simulink model "Predefined_time_v2"  (R2022a)
settings: Solver=ode8  StartTime=0  StopTime=1  FixedStep=1e-5  RelTol=1e-5
values from neighbouring files (symbols this model uses):
  order = 0.95    [predefined_time_M.m]
  phi_1 = (n*pi)/(4*Tc)    (= 47.1238898038)    [predefined_time_M.m]
  phi_2 = pi/(4*Tc)    (= 3.92699081699)    [predefined_time_M.m]
  phi_3 = (n*pi)/(4*Tc)    (= 47.1238898038)    [predefined_time_M.m]
  phi_4 = pi/(4*Tc)    (= 3.92699081699)    [predefined_time_M.m]
undefined symbols (not defined in the file or in its folder): phi_5, phi_6
libraries: cstblocks x32
(part 1 of 2)
settings Model: SimulationMode=accelerator  Creator=WIT531  LastModifiedBy=WIT531
settings SolverCC: ZeroCrossAlgorithm=Adaptive  EnableFixedStepZeroCrossing=on
settings DataIOCC: SaveFormat=Array  SaveOutput=off  SignalLogging=off  DSMLogging=off  SaveTime=off  ReturnWorkspaceOutputs=off  TimeSaveName=e2312tout  OutputSaveName=e2312
settings OptimizationCC: DefaultParameterBehavior=Inlined  EnhancedBackFolding=on  PassReuseOutputArgsAs=Individual arguments  ZeroExternalMemoryAtStartup=off  ZeroInternalMemoryAtStartup=off  InitFltsAndDblsToZero=on  OptimizeBlockOrder=speed  DifferentSizesBufferReuse=on  OptimizationCustomize=off  EfficientTunableParamExpr=on
settings DebuggingCC: ParameterTunabilityLossMsg=error
settings HardwareCC: ProdLongLongMode=on  TargetLongLongMode=on
settings SFSimCC: MATLABDynamicMemAlloc=off  SimTargetLang=C++
settings RTWCC: SystemTargetFile=ert.tlc  TemplateMakefile=ert_default_tmf  TargetLang=C++
settings CodeAppCC: ForceParamTrailComments=on  IgnoreCustomStorageClasses=off  OperatorAnnotations=on  SimulinkDataObjDesc=on  SFDataObjDesc=on  InsertBlockDesc=on
settings ERTTargetCC: TargetLangStandard=C++11 (ISO)  GenerateSampleERTMain=on  CodeInterfacePackaging=C++ class  InlinedParameterPlacement=NonHierarchical  RootIOFormat=Structure reference  ERTCustomFileTemplate=example_file_process.tlc

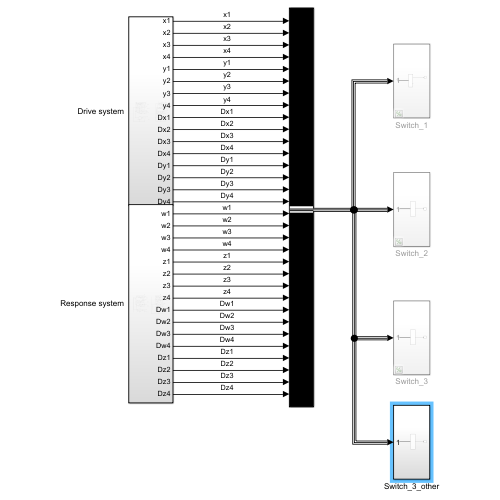
[thumbnail: Simulink's stored preview of the top-level diagram]
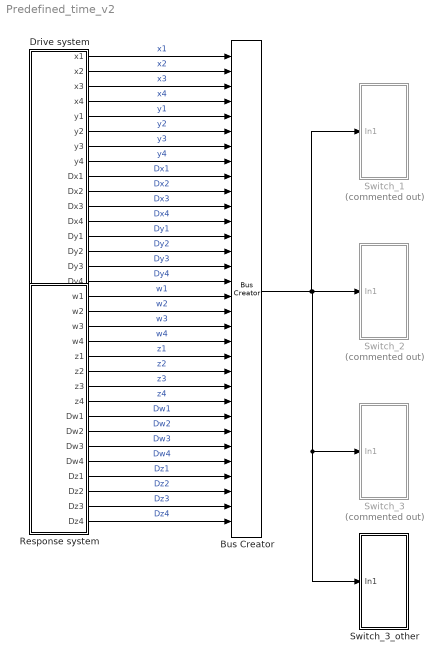
== system Predefined_time_v2 ==
  Bus Creator : BusCreator  Inputs=32
  Drive system : Subsystem
  Response system : Subsystem
  Switch_1 : Subsystem  Commented=on
  Switch_2 : Subsystem  Commented=on
  Switch_3 : Subsystem  Commented=on
  Switch_3_other : Subsystem
  wires:
  Bus Creator/1 -> Switch_3_other/1(In1), Switch_3/1(In1), Switch_2/1(In1), Switch_1/1(In1)
  Drive system/1(x1) -> Bus Creator/1  "x1"
  Drive system/2(x2) -> Bus Creator/2  "x2"
  Drive system/3(x3) -> Bus Creator/3  "x3"
  Drive system/4(x4) -> Bus Creator/4  "x4"
  Drive system/5(y1) -> Bus Creator/5  "y1"
  Drive system/6(y2) -> Bus Creator/6  "y2"
  Drive system/7(y3) -> Bus Creator/7  "y3"
  Drive system/8(y4) -> Bus Creator/8  "y4"
  Drive system/9(Dx1) -> Bus Creator/9  "Dx1"
  Drive system/10(Dx2) -> Bus Creator/10  "Dx2"
  Drive system/11(Dx3) -> Bus Creator/11  "Dx3"
  Drive system/12(Dx4) -> Bus Creator/12  "Dx4"
  Drive system/13(Dy1) -> Bus Creator/13  "Dy1"
  Drive system/14(Dy2) -> Bus Creator/14  "Dy2"
  Drive system/15(Dy3) -> Bus Creator/15  "Dy3"
  Drive system/16(Dy4) -> Bus Creator/16  "Dy4"
  Response system/9(Dw1) -> Bus Creator/25  "Dw1"
  Response system/10(Dw2) -> Bus Creator/26  "Dw2"
  Response system/11(Dw3) -> Bus Creator/27  "Dw3"
  Response system/12(Dw4) -> Bus Creator/28  "Dw4"
  Response system/13(Dz1) -> Bus Creator/29  "Dz1"
  Response system/14(Dz2) -> Bus Creator/30  "Dz2"
  Response system/15(Dz3) -> Bus Creator/31  "Dz3"
  Response system/16(Dz4) -> Bus Creator/32  "Dz4"
  Response system/1(w1) -> Bus Creator/17  "w1"
  Response system/2(w2) -> Bus Creator/18  "w2"
  Response system/3(w3) -> Bus Creator/19  "w3"
  Response system/4(w4) -> Bus Creator/20  "w4"
  Response system/5(z1) -> Bus Creator/21  "z1"
  Response system/6(z2) -> Bus Creator/22  "z2"
  Response system/7(z3) -> Bus Creator/23  "z3"
  Response system/8(z4) -> Bus Creator/24  "z4"

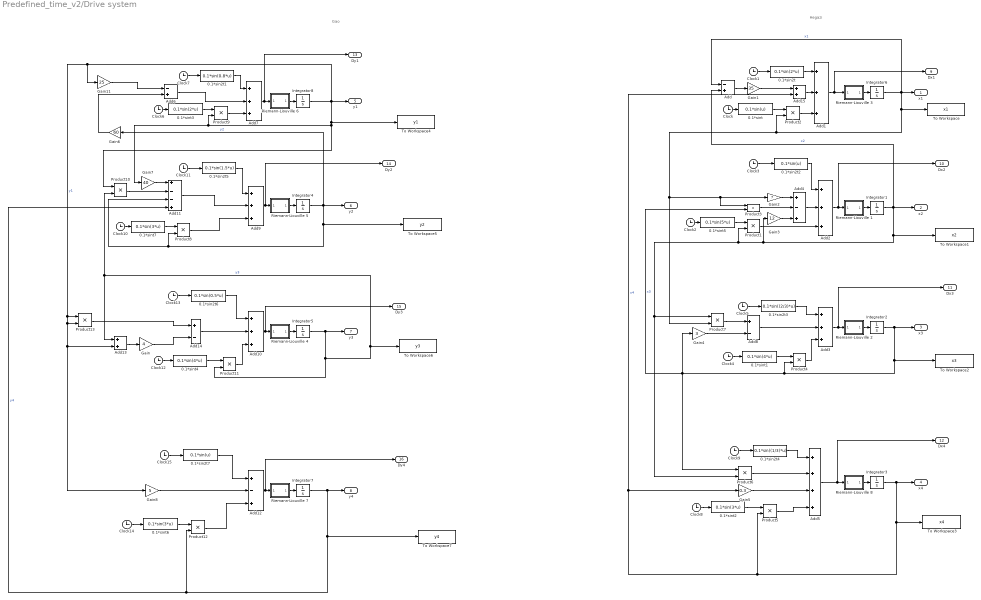
== system Predefined_time_v2/Drive system ==
  note: Gao
  note: Hegazi
  0.1*sin2t : MATLABFcn  MATLABFcn=0.1*sin(2*u)
  0.1*sin2t1 : MATLABFcn  MATLABFcn=0.1*sin(0.8*u)
  0.1*sin2t2 : MATLABFcn  MATLABFcn=0.1*sin(u)
  0.1*sin2t3 : MATLABFcn  MATLABFcn=0.1*sin((2/3)*u)
  0.1*sin2t4 : MATLABFcn  MATLABFcn=0.1*sin((1/3)*u)
  0.1*sin2t5 : MATLABFcn  MATLABFcn=0.1*sin(1.5*u)
  0.1*sin2t6 : MATLABFcn  MATLABFcn=0.1*sin(0.5*u)
  0.1*sin2t7 : MATLABFcn  MATLABFcn=0.1*sin(u)
  0.1*sint : MATLABFcn  MATLABFcn=0.1*sin(u)
  0.1*sint1 : MATLABFcn  MATLABFcn=0.1*sin(4*u)
  0.1*sint2 : MATLABFcn  MATLABFcn=0.1*sin(3*u)
  0.1*sint3 : MATLABFcn  MATLABFcn=0.1*sin(2*u)
  0.1*sint4 : MATLABFcn  MATLABFcn=0.1*sin(4*u)
  0.1*sint5 : MATLABFcn  MATLABFcn=0.1*sin(5*u)
  0.1*sint6 : MATLABFcn  MATLABFcn=0.1*sin(3*u)
  0.1*sint7 : MATLABFcn  MATLABFcn=0.1*sin(3*u)
  Add : Sum  Inputs=-+
  Add{1..3,7,9..10} (6 alike) : Sum  Inputs=+++
  Add11 : Sum  Inputs=+--+
  Add12 : Sum  Inputs=+-+
  Add13 : Sum
  Add14 : Sum  Inputs=+-
  Add15 : Sum
  Add4 : Sum  Inputs=+-+
  Add5 : Sum  Inputs=++++
  Add6 : Sum  Inputs=-+
  Add8 : Sum  Inputs=+-
  Clock{,1..15} (16 alike) : Clock
  Gain : Gain  Gain=4
  Gain1 : Gain  Gain=35
  Gain11 : Gain  Gain=25
  Gain2 : Gain  Gain=7
  Gain3 : Gain  Gain=12
  Gain4 : Gain  Gain=3
  Gain5 : Gain  Gain=0.3
  Gain6 : Gain  Gain=60
  Gain7 : Gain  Gain=40
  Gain8 : Gain  Gain=5
  Integrator{1..3,6,8} (5 alike) : Integrator  InitialCondition=10
  Integrator4 : Integrator  InitialCondition=12
  Integrator5 : Integrator  InitialCondition=15
  Integrator7 : Integrator  InitialCondition=12
  Product{1..13} (13 alike) : Product
  Riemann-Liouville 1 : Subsystem  mask{gam=1-order, ww=[1e-3, 1e3], n=5, kF1=off, kF=Oustaloup filter}
      mask prompts: gam "Derivative order gamma"; ww "Frequency range [wb,wh]"; n "Apprixmation order"; kF1 "Is a low-pass filter required?"; kF "Filter type"
      mask init:
      | wb=ww(1); wh=ww(2); 
      | if isnumeric(gam), str=['{\its}^{' num2str(gam) '}']; 
      | else, str='{\its}^{\gamma}'; end
      | if kF==1, G=ousta_fod(gam,n,wb,wh);
      | elseif kF==2, G=new_fod(gam,n,wb,wh); 
      | else, G=matsuda_fod(gam,n,wb,wh); end
      | T=1/wh; if kF1==1, G=G*tf(1,[T 1]); end
      mask TypeOptions kF: Oustaloup filter | Modified Oustaloup filter | Matsuda-Fujii filter
      mask Display: disp(str,'texmode','on')
  Riemann-Liouville 2 : Subsystem  mask{gam=1-order, ww=[1e-3, 1e3], n=5, kF1=off, kF=Oustaloup filter}
      mask prompts: gam "Derivative order gamma"; ww "Frequency range [wb,wh]"; n "Apprixmation order"; kF1 "Is a low-pass filter required?"; kF "Filter type"
      mask init: same as Predefined_time_v2/Drive system/Riemann-Liouville 1
      mask TypeOptions kF: Oustaloup filter | Modified Oustaloup filter | Matsuda-Fujii filter
      mask Display: disp(str,'texmode','on')
  Riemann-Liouville 3 : Subsystem  mask{gam=1-order, ww=[1e-3, 1e3], n=5, kF1=off, kF=Oustaloup filter}
      mask prompts: gam "Derivative order gamma"; ww "Frequency range [wb,wh]"; n "Apprixmation order"; kF1 "Is a low-pass filter required?"; kF "Filter type"
      mask init: same as Predefined_time_v2/Drive system/Riemann-Liouville 1
      mask TypeOptions kF: Oustaloup filter | Modified Oustaloup filter | Matsuda-Fujii filter
      mask Display: disp(str,'texmode','on')
  Riemann-Liouville 4 : Subsystem  mask{gam=1-order, ww=[1e-3, 1e3], n=5, kF1=off, kF=Oustaloup filter}
      mask prompts: gam "Derivative order gamma"; ww "Frequency range [wb,wh]"; n "Apprixmation order"; kF1 "Is a low-pass filter required?"; kF "Filter type"
      mask init: same as Predefined_time_v2/Drive system/Riemann-Liouville 1
      mask TypeOptions kF: Oustaloup filter | Modified Oustaloup filter | Matsuda-Fujii filter
      mask Display: disp(str,'texmode','on')
  Riemann-Liouville 5 : Subsystem  mask{gam=1-order, ww=[1e-3, 1e3], n=5, kF1=off, kF=Oustaloup filter}
      mask prompts: gam "Derivative order gamma"; ww "Frequency range [wb,wh]"; n "Apprixmation order"; kF1 "Is a low-pass filter required?"; kF "Filter type"
      mask init: same as Predefined_time_v2/Drive system/Riemann-Liouville 1
      mask TypeOptions kF: Oustaloup filter | Modified Oustaloup filter | Matsuda-Fujii filter
      mask Display: disp(str,'texmode','on')
  Riemann-Liouville 6 : Subsystem  mask{gam=1-order, ww=[1e-3, 1e3], n=5, kF1=off, kF=Oustaloup filter}
      mask prompts: gam "Derivative order gamma"; ww "Frequency range [wb,wh]"; n "Apprixmation order"; kF1 "Is a low-pass filter required?"; kF "Filter type"
      mask init: same as Predefined_time_v2/Drive system/Riemann-Liouville 1
      mask TypeOptions kF: Oustaloup filter | Modified Oustaloup filter | Matsuda-Fujii filter
      mask Display: disp(str,'texmode','on')
  Riemann-Liouville 7 : Subsystem  mask{gam=1-order, ww=[1e-3, 1e3], n=5, kF1=off, kF=Oustaloup filter}
      mask prompts: gam "Derivative order gamma"; ww "Frequency range [wb,wh]"; n "Apprixmation order"; kF1 "Is a low-pass filter required?"; kF "Filter type"
      mask init: same as Predefined_time_v2/Drive system/Riemann-Liouville 1
      mask TypeOptions kF: Oustaloup filter | Modified Oustaloup filter | Matsuda-Fujii filter
      mask Display: disp(str,'texmode','on')
  Riemann-Liouville 8 : Subsystem  mask{gam=1-order, ww=[1e-3, 1e3], n=5, kF1=off, kF=Oustaloup filter}
      mask prompts: gam "Derivative order gamma"; ww "Frequency range [wb,wh]"; n "Apprixmation order"; kF1 "Is a low-pass filter required?"; kF "Filter type"
      mask init: same as Predefined_time_v2/Drive system/Riemann-Liouville 1
      mask TypeOptions kF: Oustaloup filter | Modified Oustaloup filter | Matsuda-Fujii filter
      mask Display: disp(str,'texmode','on')
  To Workspace : ToWorkspace  VariableName=x1  SaveFormat=Timeseries  SampleTime=-1
  To Workspace1 : ToWorkspace  VariableName=x2  SaveFormat=Timeseries  SampleTime=-1
  To Workspace2 : ToWorkspace  VariableName=x3  SaveFormat=Timeseries  SampleTime=-1
  To Workspace3 : ToWorkspace  VariableName=x4  SaveFormat=Timeseries  SampleTime=-1
  To Workspace4 : ToWorkspace  VariableName=y1  SaveFormat=Timeseries  SampleTime=-1
  To Workspace5 : ToWorkspace  VariableName=y2  SaveFormat=Timeseries  SampleTime=-1
  To Workspace6 : ToWorkspace  VariableName=y3  SaveFormat=Timeseries  SampleTime=-1
  To Workspace7 : ToWorkspace  VariableName=y4  SaveFormat=Timeseries  SampleTime=-1
  x1 : Outport
  x2 : Outport  Port=2
  x3 : Outport  Port=3
  x4 : Outport  Port=4
  y1 : Outport  Port=5
  y2 : Outport  Port=6
  y3 : Outport  Port=7
  y4 : Outport  Port=8
  Dx1 : Outport  Port=9
  Dx2 : Outport  Port=10
  Dx3 : Outport  Port=11
  Dx4 : Outport  Port=12
  Dy1 : Outport  Port=13
  Dy2 : Outport  Port=14
  Dy3 : Outport  Port=15
  Dy4 : Outport  Port=16
  wires:
  Integrator6/1 -> Add/1, x1/1, To Workspace/1, Product2/2, Product7/2, Product3/1, Gain2/1  "x1"
  Add1/1 -> Riemann-Liouville 3/1(In1), Dx1/1
  0.1*sint/1 -> Product2/1
  Clock/1 -> 0.1*sint/1
  Clock1/1 -> 0.1*sin2t/1
  Add2/1 -> Riemann-Liouville 1/1(In1), Dx2/1
  Add/1 -> Gain1/1
  Gain1/1 -> Add15/1
  0.1*sint5/1 -> Product1/1
  Integrator1/1 -> Add/2, x2/1, To Workspace1/1, Product7/1, Product6/2, Product1/2, Gain3/1  "x2"
  Clock2/1 -> 0.1*sint5/1
  Clock3/1 -> 0.1*sin2t2/1
  Gain2/1 -> Add4/1
  Integrator2/1 -> To Workspace2/1, Product6/1, Gain4/1, Product3/2, Product4/2, x3/1  "x3"
  Add3/1 -> Riemann-Liouville 2/1(In1), Dx3/1
  Add4/1 -> Add2/2
  Add5/1 -> Riemann-Liouville 8/1(In1), Dx4/1
  Integrator3/1 -> To Workspace3/1, Gain5/1, Add15/2, Product5/2, x4/1  "x4"
  Clock4/1 -> 0.1*sint1/1
  0.1*sint1/1 -> Product4/1
  Add8/1 -> Add3/2
  Clock5/1 -> 0.1*sin2t3/1
  Product6/1 -> Add5/2
  Gain5/1 -> Add5/3
  Clock8/1 -> 0.1*sint2/1
  0.1*sint2/1 -> Product5/1
  Clock9/1 -> 0.1*sin2t4/1
  Product7/1 -> Add8/1
  Clock13/1 -> 0.1*sin2t6/1
  Clock12/1 -> 0.1*sint4/1
  Integrator7/1 -> To Workspace7/1, Add11/4, Product12/2, y4/1  "y4"
  Add12/1 -> Riemann-Liouville 7/1(In1), Dy4/1
  Add10/1 -> Riemann-Liouville 4/1(In1), Dy3/1
  Clock14/1 -> 0.1*sint6/1
  0.1*sint7/1 -> Product8/1
  Clock10/1 -> 0.1*sint7/1
  Clock7/1 -> 0.1*sin2t1/1
  0.1*sint3/1 -> Product9/1
  Clock11/1 -> 0.1*sin2t5/1
  Clock6/1 -> 0.1*sint3/1
  Integrator8/1 -> Gain11/1, Add13/2, Gain8/1, Product13/2, Product13/1, y1/1, To Workspace4/1, Product10/1, Gain7/1, Product9/2  "y1"
  Add6/1 -> Add7/2
  Integrator5/1 -> To Workspace6/1, Add13/1, Product10/2, Product11/2, y3/1  "y3"
  Add7/1 -> Riemann-Liouville 6/1(In1), Dy1/1
  0.1*sint4/1 -> Product11/1
  Clock15/1 -> 0.1*sin2t7/1
  0.1*sint6/1 -> Product12/1
  Add9/1 -> Riemann-Liouville 5/1(In1), Dy2/1
  Riemann-Liouville 7/1(Out1) -> Integrator7/1
  Add11/1 -> Add9/2
  Add13/1 -> Gain/1
  Product13/1 -> Add14/1
  Gain/1 -> Add14/2
  Add14/1 -> Add10/2
  Gain8/1 -> Add12/2
  Add15/1 -> Add1/2
  Product3/1 -> Add4/2
  Gain3/1 -> Add4/3
  Gain7/1 -> Add11/1
  Product10/1 -> Add11/2
  Integrator4/1 -> Gain6/1, To Workspace5/1, Add11/3, Product8/2, y2/1  "y2"
  Riemann-Liouville 6/1(Out1) -> Integrator8/1
  Riemann-Liouville 5/1(Out1) -> Integrator4/1
  Riemann-Liouville 4/1(Out1) -> Integrator5/1
  Riemann-Liouville 3/1(Out1) -> Integrator6/1
  Riemann-Liouville 1/1(Out1) -> Integrator1/1
  Riemann-Liouville 2/1(Out1) -> Integrator2/1
  Riemann-Liouville 8/1(Out1) -> Integrator3/1
  0.1*sin2t1/1 -> Add7/1
  Product9/1 -> Add7/3
  0.1*sin2t5/1 -> Add9/1
  Product8/1 -> Add9/3
  0.1*sin2t6/1 -> Add10/1
  Product11/1 -> Add10/3
  0.1*sin2t7/1 -> Add12/1
  Product12/1 -> Add12/3
  Product5/1 -> Add5/4
  0.1*sin2t4/1 -> Add5/1
  Product4/1 -> Add3/3
  0.1*sin2t3/1 -> Add3/1
  0.1*sin2t2/1 -> Add2/1
  Product1/1 -> Add2/3
  Product2/1 -> Add1/3
  0.1*sin2t/1 -> Add1/1
  Gain4/1 -> Add8/2
  Gain11/1 -> Add6/1
  Gain6/1 -> Add6/2

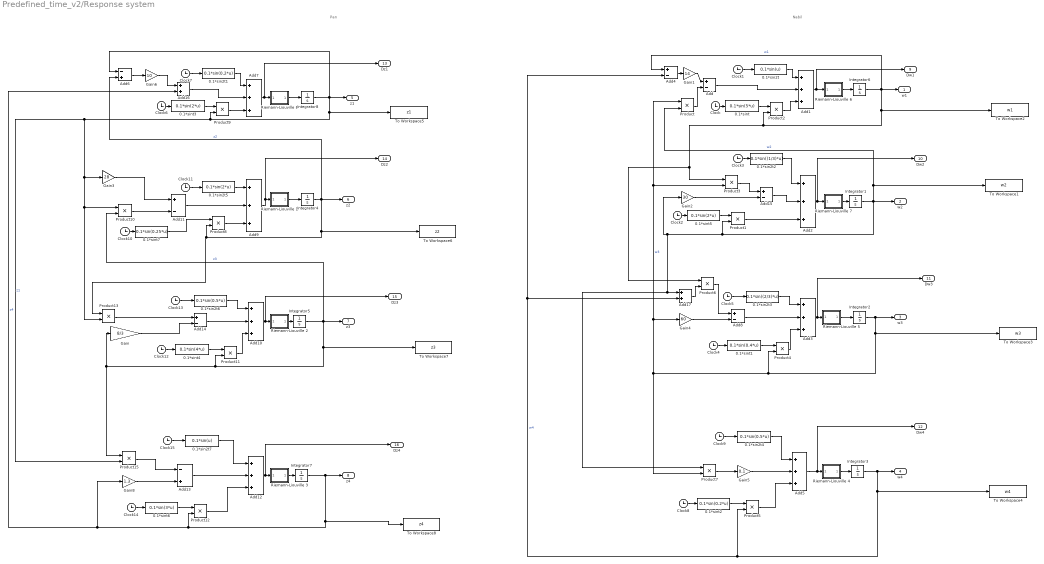
== system Predefined_time_v2/Response system ==
  note: Pan
  note: Nabil
  0.1*sin2t : MATLABFcn  MATLABFcn=0.1*sin(u)
  0.1*sin2t1 : MATLABFcn  MATLABFcn=0.1*sin(0.2*u)
  0.1*sin2t2 : MATLABFcn  MATLABFcn=0.1*sin((1/3)*u)
  0.1*sin2t3 : MATLABFcn  MATLABFcn=0.1*sin((2/3)*u)
  0.1*sin2t4 : MATLABFcn  MATLABFcn=0.1*sin(0.5*u)
  0.1*sin2t5 : MATLABFcn  MATLABFcn=0.1*sin(2*u)
  0.1*sin2t6 : MATLABFcn  MATLABFcn=0.1*sin(0.5*u)
  0.1*sin2t7 : MATLABFcn  MATLABFcn=0.1*sin(u)
  0.1*sint : MATLABFcn  MATLABFcn=0.1*sin(5*u)
  0.1*sint1 : MATLABFcn  MATLABFcn=0.1*sin(0.4*u)
  0.1*sint2 : MATLABFcn  MATLABFcn=0.1*sin(0.2*u)
  0.1*sint3 : MATLABFcn  MATLABFcn=0.1*sin(2*u)
  0.1*sint4 : MATLABFcn  MATLABFcn=0.1*sin(4*u)
  0.1*sint5 : MATLABFcn  MATLABFcn=0.1*sin(2*u)
  0.1*sint6 : MATLABFcn  MATLABFcn=0.1*sin(3*u)
  0.1*sint7 : MATLABFcn  MATLABFcn=0.1*sin(0.25*u)
  Add{,4,8,11,14..15} (6 alike) : Sum  Inputs=+-
  Add{1..3,5,7,9..10,12} (8 alike) : Sum  Inputs=+++
  Add13 : Sum  Inputs=-+
  Add16 : Sum
  Add17 : Sum
  Add6 : Sum  Inputs=-+
  Clock{,1..15} (16 alike) : Clock
  Gain : Gain  Gain=8/3
  Gain1 : Gain  Gain=14
  Gain2 : Gain  Gain=30
  Gain3 : Gain  Gain=28
  Gain4 : Gain  Gain=60
  Gain5 : Gain  Gain=0.1
  Gain6 : Gain  Gain=10
  Gain8 : Gain  Gain=1.3
  Integrator1 : Integrator  InitialCondition=14
  Integrator2 : Integrator  InitialCondition=12
  Integrator3 : Integrator  InitialCondition=13
  Integrator4 : Integrator  InitialCondition=3
  Integrator5 : Integrator  InitialCondition=16
  Integrator6 : Integrator  InitialCondition=21
  Integrator7 : Integrator  InitialCondition=17
  Integrator8 : Integrator  InitialCondition=15
  Product{,1..13,15} (15 alike) : Product
  Riemann-Liouville 1 : Subsystem  mask{gam=1-order, ww=[1e-3, 1e3], n=5, kF1=off, kF=Oustaloup filter}
      mask prompts: gam "Derivative order gamma"; ww "Frequency range [wb,wh]"; n "Apprixmation order"; kF1 "Is a low-pass filter required?"; kF "Filter type"
      mask init: same as Predefined_time_v2/Drive system/Riemann-Liouville 1
      mask TypeOptions kF: Oustaloup filter | Modified Oustaloup filter | Matsuda-Fujii filter
      mask Display: disp(str,'texmode','on')
  Riemann-Liouville 2 : Subsystem  mask{gam=1-order, ww=[1e-3, 1e3], n=5, kF1=off, kF=Oustaloup filter}
      mask prompts: gam "Derivative order gamma"; ww "Frequency range [wb,wh]"; n "Apprixmation order"; kF1 "Is a low-pass filter required?"; kF "Filter type"
      mask init: same as Predefined_time_v2/Drive system/Riemann-Liouville 1
      mask TypeOptions kF: Oustaloup filter | Modified Oustaloup filter | Matsuda-Fujii filter
      mask Display: disp(str,'texmode','on')
  Riemann-Liouville 3 : Subsystem  mask{gam=1-order, ww=[1e-3, 1e3], n=5, kF1=off, kF=Oustaloup filter}
      mask prompts: gam "Derivative order gamma"; ww "Frequency range [wb,wh]"; n "Apprixmation order"; kF1 "Is a low-pass filter required?"; kF "Filter type"
      mask init: same as Predefined_time_v2/Drive system/Riemann-Liouville 1
      mask TypeOptions kF: Oustaloup filter | Modified Oustaloup filter | Matsuda-Fujii filter
      mask Display: disp(str,'texmode','on')
  Riemann-Liouville 4 : Subsystem  mask{gam=1-order, ww=[1e-3, 1e3], n=5, kF1=off, kF=Oustaloup filter}
      mask prompts: gam "Derivative order gamma"; ww "Frequency range [wb,wh]"; n "Apprixmation order"; kF1 "Is a low-pass filter required?"; kF "Filter type"
      mask init: same as Predefined_time_v2/Drive system/Riemann-Liouville 1
      mask TypeOptions kF: Oustaloup filter | Modified Oustaloup filter | Matsuda-Fujii filter
      mask Display: disp(str,'texmode','on')
  Riemann-Liouville 5 : Subsystem  mask{gam=1-order, ww=[1e-3, 1e3], n=5, kF1=off, kF=Oustaloup filter}
      mask prompts: gam "Derivative order gamma"; ww "Frequency range [wb,wh]"; n "Apprixmation order"; kF1 "Is a low-pass filter required?"; kF "Filter type"
      mask init: same as Predefined_time_v2/Drive system/Riemann-Liouville 1
      mask TypeOptions kF: Oustaloup filter | Modified Oustaloup filter | Matsuda-Fujii filter
      mask Display: disp(str,'texmode','on')
  Riemann-Liouville 6 : Subsystem  mask{gam=1-order, ww=[1e-3, 1e3], n=5, kF1=off, kF=Oustaloup filter}
      mask prompts: gam "Derivative order gamma"; ww "Frequency range [wb,wh]"; n "Apprixmation order"; kF1 "Is a low-pass filter required?"; kF "Filter type"
      mask init: same as Predefined_time_v2/Drive system/Riemann-Liouville 1
      mask TypeOptions kF: Oustaloup filter | Modified Oustaloup filter | Matsuda-Fujii filter
      mask Display: disp(str,'texmode','on')
  Riemann-Liouville 7 : Subsystem  mask{gam=1-order, ww=[1e-3, 1e3], n=5, kF1=off, kF=Oustaloup filter}
      mask prompts: gam "Derivative order gamma"; ww "Frequency range [wb,wh]"; n "Apprixmation order"; kF1 "Is a low-pass filter required?"; kF "Filter type"
      mask init: same as Predefined_time_v2/Drive system/Riemann-Liouville 1
      mask TypeOptions kF: Oustaloup filter | Modified Oustaloup filter | Matsuda-Fujii filter
      mask Display: disp(str,'texmode','on')
  Riemann-Liouville 8 : Subsystem  mask{gam=1-order, ww=[1e-3, 1e3], n=5, kF1=off, kF=Oustaloup filter}
      mask prompts: gam "Derivative order gamma"; ww "Frequency range [wb,wh]"; n "Apprixmation order"; kF1 "Is a low-pass filter required?"; kF "Filter type"
      mask init: same as Predefined_time_v2/Drive system/Riemann-Liouville 1
      mask TypeOptions kF: Oustaloup filter | Modified Oustaloup filter | Matsuda-Fujii filter
      mask Display: disp(str,'texmode','on')
  To Workspace1 : ToWorkspace  VariableName=w2  SaveFormat=Timeseries  SampleTime=-1
  To Workspace2 : ToWorkspace  VariableName=w1  SaveFormat=Timeseries  SampleTime=-1
  To Workspace3 : ToWorkspace  VariableName=w3  SaveFormat=Timeseries  SampleTime=-1
  To Workspace4 : ToWorkspace  VariableName=w4  SaveFormat=Timeseries  SampleTime=-1
  To Workspace5 : ToWorkspace  VariableName=z1  SaveFormat=Timeseries  SampleTime=-1
  To Workspace6 : ToWorkspace  VariableName=z2  SaveFormat=Timeseries  SampleTime=-1
  To Workspace7 : ToWorkspace  VariableName=z3  SaveFormat=Timeseries  SampleTime=-1
  To Workspace8 : ToWorkspace  VariableName=z4  SaveFormat=Timeseries  SampleTime=-1
  w1 : Outport
  w2 : Outport  Port=2
  w3 : Outport  Port=3
  w4 : Outport  Port=4
  z1 : Outport  Port=5
  z2 : Outport  Port=6
  z3 : Outport  Port=7
  z4 : Outport  Port=8
  Dw1 : Outport  Port=9
  Dw2 : Outport  Port=10
  Dw3 : Outport  Port=11
  Dw4 : Outport  Port=12
  Dz1 : Outport  Port=13
  Dz2 : Outport  Port=14
  Dz3 : Outport  Port=15
  Dz4 : Outport  Port=16
  wires:
  Integrator6/1 -> Add4/1, To Workspace2/1, Product2/2, Product3/1, Product6/1, w1/1  "w1"
  Add1/1 -> Riemann-Liouville 6/1(In1), Dw1/1
  Riemann-Liouville 6/1(Out1) -> Integrator6/1
  0.1*sint/1 -> Product2/1
  Clock/1 -> 0.1*sint/1
  Clock1/1 -> 0.1*sin2t/1
  Add2/1 -> Riemann-Liouville 7/1(In1), Dw2/1
  Riemann-Liouville 7/1(Out1) -> Integrator1/1
  0.1*sint5/1 -> Product1/1
  Integrator1/1 -> To Workspace1/1, Product/2, Product1/2, Add17/1, Product7/1, Gain2/1, w2/1  "w2"
  Clock2/1 -> 0.1*sint5/1
  Clock3/1 -> 0.1*sin2t2/1
  Integrator2/1 -> To Workspace3/1, Product3/2, Product/1, Gain4/1, Product7/2, Product4/2, w3/1  "w3"
  Riemann-Liouville 5/1(Out1) -> Integrator2/1
  Add3/1 -> Riemann-Liouville 5/1(In1), Dw3/1
  Add5/1 -> Riemann-Liouville 4/1(In1), Dw4/1
  Integrator3/1 -> To Workspace4/1, Product5/2, Add17/2, Add4/2, w4/1  "w4"
  Riemann-Liouville 4/1(Out1) -> Integrator3/1
  Clock4/1 -> 0.1*sint1/1
  0.1*sint1/1 -> Product4/1
  Clock5/1 -> 0.1*sin2t3/1
  Clock8/1 -> 0.1*sint2/1
  0.1*sint2/1 -> Product5/1
  Clock9/1 -> 0.1*sin2t4/1
  Clock13/1 -> 0.1*sin2t6/1
  Clock12/1 -> 0.1*sint4/1
  Integrator7/1 -> To Workspace8/1, Gain8/1, Add16/2, Product12/2, z4/1  "z4"
  Add12/1 -> Riemann-Liouville 3/1(In1), Dz4/1
  Add10/1 -> Riemann-Liouville 2/1(In1), Dz3/1
  Clock14/1 -> 0.1*sint6/1
  Integrator4/1 -> Add6/2, Product13/1, Product8/2, To Workspace6/1, z2/1  "z2"
  0.1*sint7/1 -> Product8/1
  Clock10/1 -> 0.1*sint7/1
  Clock7/1 -> 0.1*sin2t1/1
  0.1*sint3/1 -> Product9/1
  Clock11/1 -> 0.1*sin2t5/1
  Clock6/1 -> 0.1*sint3/1
  Integrator8/1 -> Add6/1, z1/1, To Workspace5/1, Gain3/1, Product13/2, Product10/1, Product15/2, Product9/2  "z1"
  Add16/1 -> Add7/2
  Integrator5/1 -> Product10/2, To Workspace7/1, Product15/1, Gain/1, Product11/2, z3/1  "z3"
  Add7/1 -> Riemann-Liouville 8/1(In1), Dz1/1
  0.1*sint4/1 -> Product11/1
  Clock15/1 -> 0.1*sin2t7/1
  0.1*sint6/1 -> Product12/1
  Add9/1 -> Riemann-Liouville 1/1(In1), Dz2/1
  Product13/1 -> Add14/1
  Add14/1 -> Add10/2
  Gain8/1 -> Add13/2
  Product7/1 -> Gain5/1
  Add6/1 -> Gain6/1
  Product10/1 -> Add11/2
  Gain3/1 -> Add11/1
  Add11/1 -> Add9/2
  Add13/1 -> Add12/2
  Product15/1 -> Add13/1
  Gain6/1 -> Add16/1
  Riemann-Liouville 8/1(Out1) -> Integrator8/1
  Riemann-Liouville 1/1(Out1) -> Integrator4/1
  Riemann-Liouville 2/1(Out1) -> Integrator5/1
  Riemann-Liouville 3/1(Out1) -> Integrator7/1
  0.1*sin2t1/1 -> Add7/1
  Product9/1 -> Add7/3
  0.1*sin2t5/1 -> Add9/1
  Product8/1 -> Add9/3
  0.1*sin2t6/1 -> Add10/1
  Product11/1 -> Add10/3
  Product12/1 -> Add12/3
  0.1*sin2t7/1 -> Add12/1
  0.1*sin2t/1 -> Add1/1
  Product2/1 -> Add1/3
  0.1*sin2t2/1 -> Add2/1
  Product1/1 -> Add2/3
  Product4/1 -> Add3/3
  0.1*sin2t3/1 -> Add3/1
  0.1*sin2t4/1 -> Add5/1
  Product5/1 -> Add5/3
  Product/1 -> Add/2
  Add4/1 -> Gain1/1
  Gain1/1 -> Add/1
  Add/1 -> Add1/2
  Product3/1 -> Add15/1
  Gain2/1 -> Add15/2
  Add15/1 -> Add2/2
  Add17/1 -> Product6/2
  Product6/1 -> Add8/1
  Add8/1 -> Add3/2
  Gain5/1 -> Add5/2
  Gain/1 -> Add14/2
  Gain4/1 -> Add8/2

== system Predefined_time_v2/Switch_1 ==
  In1 : Inport
  Scope : Scope
  e3142 : Subsystem
  wires:
  In1/1 -> e3142/1(In1)
  e3142/1(error) -> Scope/1

== system Predefined_time_v2/Switch_2 ==
  In1 : Inport
  Scope : Scope
  e2314 : Subsystem
  wires:
  In1/1 -> e2314/1(In1)
  e2314/1(error) -> Scope/1

== system Predefined_time_v2/Switch_3 ==
  In1 : Inport
  Scope : Scope
  e3421 : Subsystem
  wires:
  In1/1 -> e3421/1(In1)
  e3421/1(error) -> Scope/1

== system Predefined_time_v2/Switch_3_other ==
  In1 : Inport
  Scope : Scope
  e3421 : Subsystem
  wires:
  In1/1 -> e3421/1(In1)
  e3421/1(error) -> Scope/1

== system Predefined_time_v2/Drive system/Riemann-Liouville 1 ==
  In1 : Inport
  LTI System : cstblocks/LTI System  sys=G  IC=[]
  Out1 : Outport
  wires:
  In1/1 -> LTI System/1
  LTI System/1 -> Out1/1

== system Predefined_time_v2/Drive system/Riemann-Liouville 2 ==
  In1 : Inport
  LTI System : cstblocks/LTI System  sys=G  IC=[]
  Out1 : Outport
  wires:
  In1/1 -> LTI System/1
  LTI System/1 -> Out1/1

== system Predefined_time_v2/Drive system/Riemann-Liouville 3 ==
  In1 : Inport
  LTI System : cstblocks/LTI System  sys=G  IC=[]
  Out1 : Outport
  wires:
  In1/1 -> LTI System/1
  LTI System/1 -> Out1/1

== system Predefined_time_v2/Drive system/Riemann-Liouville 4 ==
  In1 : Inport
  LTI System : cstblocks/LTI System  sys=G  IC=[]
  Out1 : Outport
  wires:
  In1/1 -> LTI System/1
  LTI System/1 -> Out1/1

== system Predefined_time_v2/Drive system/Riemann-Liouville 5 ==
  In1 : Inport
  LTI System : cstblocks/LTI System  sys=G  IC=[]
  Out1 : Outport
  wires:
  In1/1 -> LTI System/1
  LTI System/1 -> Out1/1

== system Predefined_time_v2/Drive system/Riemann-Liouville 6 ==
  In1 : Inport
  LTI System : cstblocks/LTI System  sys=G  IC=[]
  Out1 : Outport
  wires:
  In1/1 -> LTI System/1
  LTI System/1 -> Out1/1

== system Predefined_time_v2/Drive system/Riemann-Liouville 7 ==
  In1 : Inport
  LTI System : cstblocks/LTI System  sys=G  IC=[]
  Out1 : Outport
  wires:
  In1/1 -> LTI System/1
  LTI System/1 -> Out1/1

== system Predefined_time_v2/Drive system/Riemann-Liouville 8 ==
  In1 : Inport
  LTI System : cstblocks/LTI System  sys=G  IC=[]
  Out1 : Outport
  wires:
  In1/1 -> LTI System/1
  LTI System/1 -> Out1/1

== system Predefined_time_v2/Response system/Riemann-Liouville 1 ==
  In1 : Inport
  LTI System : cstblocks/LTI System  sys=G  IC=[]
  Out1 : Outport
  wires:
  In1/1 -> LTI System/1
  LTI System/1 -> Out1/1

== system Predefined_time_v2/Response system/Riemann-Liouville 2 ==
  In1 : Inport
  LTI System : cstblocks/LTI System  sys=G  IC=[]
  Out1 : Outport
  wires:
  In1/1 -> LTI System/1
  LTI System/1 -> Out1/1

== system Predefined_time_v2/Response system/Riemann-Liouville 3 ==
  In1 : Inport
  LTI System : cstblocks/LTI System  sys=G  IC=[]
  Out1 : Outport
  wires:
  In1/1 -> LTI System/1
  LTI System/1 -> Out1/1

== system Predefined_time_v2/Response system/Riemann-Liouville 4 ==
  In1 : Inport
  LTI System : cstblocks/LTI System  sys=G  IC=[]
  Out1 : Outport
  wires:
  In1/1 -> LTI System/1
  LTI System/1 -> Out1/1

== system Predefined_time_v2/Response system/Riemann-Liouville 5 ==
  In1 : Inport
  LTI System : cstblocks/LTI System  sys=G  IC=[]
  Out1 : Outport
  wires:
  In1/1 -> LTI System/1
  LTI System/1 -> Out1/1

== system Predefined_time_v2/Response system/Riemann-Liouville 6 ==
  In1 : Inport
  LTI System : cstblocks/LTI System  sys=G  IC=[]
  Out1 : Outport
  wires:
  In1/1 -> LTI System/1
  LTI System/1 -> Out1/1

== system Predefined_time_v2/Response system/Riemann-Liouville 7 ==
  In1 : Inport
  LTI System : cstblocks/LTI System  sys=G  IC=[]
  Out1 : Outport
  wires:
  In1/1 -> LTI System/1
  LTI System/1 -> Out1/1

== system Predefined_time_v2/Response system/Riemann-Liouville 8 ==
  In1 : Inport
  LTI System : cstblocks/LTI System  sys=G  IC=[]
  Out1 : Outport
  wires:
  In1/1 -> LTI System/1
  LTI System/1 -> Out1/1

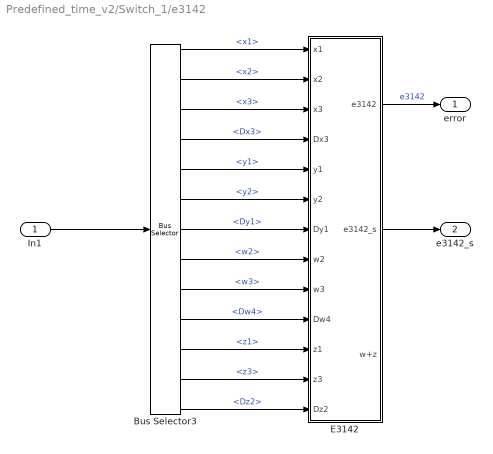
== system Predefined_time_v2/Switch_1/e3142 ==
  In1 : Inport
  Bus Selector3 : BusSelector  OutputSignals=x1,x2,x3,Dx3,y1,y2,Dy1,w2,w3,Dw4,z1,z3,Dz2
  E3142 : Subsystem
  error : Outport
  e3142_s : Outport  Port=2
  wires:
  In1/1 -> Bus Selector3/1
  E3142/1(e3142) -> error/1  "e3142"
  E3142/2(e3142_s) -> e3142_s/1
  Bus Selector3/2 -> E3142/2(x2)  "<x2>"
  Bus Selector3/3 -> E3142/3(x3)  "<x3>"
  Bus Selector3/4 -> E3142/4(Dx3)  "<Dx3>"
  Bus Selector3/6 -> E3142/6(y2)  "<y2>"
  Bus Selector3/5 -> E3142/5(y1)  "<y1>"
  Bus Selector3/7 -> E3142/7(Dy1)  "<Dy1>"
  Bus Selector3/8 -> E3142/8(w2)  "<w2>"
  Bus Selector3/9 -> E3142/9(w3)  "<w3>"
  Bus Selector3/10 -> E3142/10(Dw4)  "<Dw4>"
  Bus Selector3/11 -> E3142/11(z1)  "<z1>"
  Bus Selector3/12 -> E3142/12(z3)  "<z3>"
  Bus Selector3/13 -> E3142/13(Dz2)  "<Dz2>"
  Bus Selector3/1 -> E3142/1(x1)  "<x1>"

== system Predefined_time_v2/Switch_2/e2314 ==
  In1 : Inport
  Bus Selector3 : BusSelector  OutputSignals=x1,x2,x3,Dx2,y1,y3,Dy3,w1,w2,w3,w4,Dw1,z1,z3,z4,Dz4
  E2314 : Subsystem
  error : Outport
  wires:
  In1/1 -> Bus Selector3/1
  E2314/1(e2314) -> error/1  "e3142"
  Bus Selector3/1 -> E2314/1(x1)  "<x1>"
  Bus Selector3/2 -> E2314/2(x2)  "<x2>"
  Bus Selector3/3 -> E2314/3(x3)  "<x3>"
  Bus Selector3/4 -> E2314/4(Dx2)  "<Dx2>"
  Bus Selector3/5 -> E2314/5(y1)  "<y1>"
  Bus Selector3/7 -> E2314/7(Dy3)  "<Dy3>"
  Bus Selector3/6 -> E2314/6(y3)  "<y3>"
  Bus Selector3/8 -> E2314/8(w1)  "<w1>"
  Bus Selector3/12 -> E2314/12(Dw1)  "<Dw1>"
  Bus Selector3/13 -> E2314/13(z1)  "<z1>"
  Bus Selector3/14 -> E2314/14(z3)  "<z3>"
  Bus Selector3/15 -> E2314/15(z4)  "<z4>"
  Bus Selector3/16 -> E2314/16(Dz4)  "<Dz4>"
  Bus Selector3/9 -> E2314/9(w2)  "<w2>"
  Bus Selector3/11 -> E2314/11(w4)  "<w4>"
  Bus Selector3/10 -> E2314/10(w3)  "<w3>"

== system Predefined_time_v2/Switch_3/e3421 ==
  In1 : Inport
  Bus Selector3 : BusSelector  OutputSignals=x2,x3,x4,Dx4,y1,y3,Dy3,w1,w2,w3,Dw2,z1,z2,z4,Dz1
  E4321 : Subsystem
  error : Outport
  wires:
  In1/1 -> Bus Selector3/1
  E4321/1(e4321) -> error/1  "e4321"
  Bus Selector3/1 -> E4321/1(x2)  "<x2>"
  Bus Selector3/2 -> E4321/2(x3)  "<x3>"
  Bus Selector3/8 -> E4321/8(w1)  "<w1>"
  Bus Selector3/12 -> E4321/12(z1)  "<z1>"
  Bus Selector3/13 -> E4321/13(z2)  "<z2>"
  Bus Selector3/14 -> E4321/14(z4)  "<z4>"
  Bus Selector3/9 -> E4321/9(w2)  "<w2>"
  Bus Selector3/10 -> E4321/10(w3)  "<w3>"
  Bus Selector3/15 -> E4321/15(Dz1)  "<Dz1>"
  Bus Selector3/11 -> E4321/11(Dw2)  "<Dw2>"
  Bus Selector3/3 -> E4321/3(x4)  "<x4>"
  Bus Selector3/4 -> E4321/4(Dx4)  "<Dx4>"
  Bus Selector3/5 -> E4321/5(y1)  "<y1>"
  Bus Selector3/6 -> E4321/6(y3)  "<y3>"
  Bus Selector3/7 -> E4321/7(Dy3)  "<Dy3>"

== system Predefined_time_v2/Switch_3_other/e3421 ==
  In1 : Inport
  Bus Selector3 : BusSelector  OutputSignals=x2,x3,x4,Dx4,y1,y3,Dy3,w1,w2,w3,Dw2,z1,z2,z4,Dz1
  E4321 : Subsystem
  error : Outport
  wires:
  In1/1 -> Bus Selector3/1
  E4321/1(e4321) -> error/1  "e4321"
  Bus Selector3/1 -> E4321/1(x2)  "<x2>"
  Bus Selector3/2 -> E4321/2(x3)  "<x3>"
  Bus Selector3/8 -> E4321/8(w1)  "<w1>"
  Bus Selector3/12 -> E4321/12(z1)  "<z1>"
  Bus Selector3/13 -> E4321/13(z2)  "<z2>"
  Bus Selector3/14 -> E4321/14(z4)  "<z4>"
  Bus Selector3/9 -> E4321/9(w2)  "<w2>"
  Bus Selector3/10 -> E4321/10(w3)  "<w3>"
  Bus Selector3/15 -> E4321/15(Dz1)  "<Dz1>"
  Bus Selector3/11 -> E4321/11(Dw2)  "<Dw2>"
  Bus Selector3/3 -> E4321/3(x4)  "<x4>"
  Bus Selector3/4 -> E4321/4(Dx4)  "<Dx4>"
  Bus Selector3/5 -> E4321/5(y1)  "<y1>"
  Bus Selector3/6 -> E4321/6(y3)  "<y3>"
  Bus Selector3/7 -> E4321/7(Dy3)  "<Dy3>"

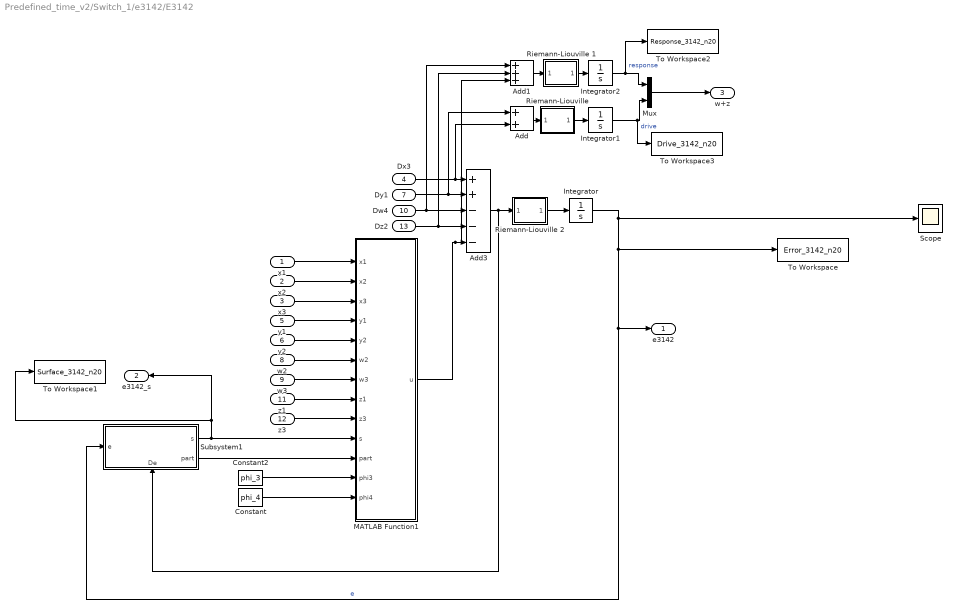
== system Predefined_time_v2/Switch_1/e3142/E3142 ==
  x1 : Inport
  x2 : Inport  Port=2
  x3 : Inport  Port=3
  Dx3 : Inport  Port=4
  y1 : Inport  Port=5
  y2 : Inport  Port=6
  Dy1 : Inport  Port=7
  w2 : Inport  Port=8
  w3 : Inport  Port=9
  Dw4 : Inport  Port=10
  z1 : Inport  Port=11
  z3 : Inport  Port=12
  Dz2 : Inport  Port=13
  Add : Sum
  Add1 : Sum  Inputs=+++
  Add3 : Sum  Inputs=++---
  Constant : Constant  Value=phi_4
  Constant2 : Constant  Value=phi_3
  Integrator : Integrator  InitialCondition=0.05
  Integrator1 : Integrator
  Integrator2 : Integrator
  MATLAB Function1 : MATLAB Function  TreatAsAtomicUnit=on
  Mux : Mux  Inputs=2
  "Riemann-Liouville " : Subsystem  mask{gam=1-order, ww=[1e-3, 1e3], n=5, kF1=off, kF=Oustaloup filter}
      mask prompts: gam "Derivative order gamma"; ww "Frequency range [wb,wh]"; n "Apprixmation order"; kF1 "Is a low-pass filter required?"; kF "Filter type"
      mask init: same as Predefined_time_v2/Drive system/Riemann-Liouville 1
      mask TypeOptions kF: Oustaloup filter | Modified Oustaloup filter | Matsuda-Fujii filter
      mask Display: disp(str,'texmode','on')
  Riemann-Liouville 1 : Subsystem  mask{gam=1-order, ww=[1e-3, 1e3], n=5, kF1=off, kF=Oustaloup filter}
      mask prompts: gam "Derivative order gamma"; ww "Frequency range [wb,wh]"; n "Apprixmation order"; kF1 "Is a low-pass filter required?"; kF "Filter type"
      mask init: same as Predefined_time_v2/Drive system/Riemann-Liouville 1
      mask TypeOptions kF: Oustaloup filter | Modified Oustaloup filter | Matsuda-Fujii filter
      mask Display: disp(str,'texmode','on')
  Riemann-Liouville 2 : Subsystem  mask{gam=1-order, ww=[1e-3, 1e3], n=5, kF1=off, kF=Oustaloup filter}
      mask prompts: gam "Derivative order gamma"; ww "Frequency range [wb,wh]"; n "Apprixmation order"; kF1 "Is a low-pass filter required?"; kF "Filter type"
      mask init: same as Predefined_time_v2/Drive system/Riemann-Liouville 1
      mask TypeOptions kF: Oustaloup filter | Modified Oustaloup filter | Matsuda-Fujii filter
      mask Display: disp(str,'texmode','on')
  Scope : Scope
  Subsystem1 : Subsystem
      settings: PortSchema="{\"entries\":[{\"content\":{\"sides\":[{\"content\":{\"connectorIds\":[\"In1\"]},\"type\":\"ConnectorPlacement.EquallySpacedRectSide\",\"uuid\":\"1e5d287b-80a1-40a3-bd98-2fb678fb874f\"},{\"content\":{\"connectorIds\":[\"Out1\",\"Out2\"],\"side\":\"RIGHT\"},\"type\":\"ConnectorPlacement.EquallySpacedRectSide\",\"uuid\":\"9f557e7f-4584-4da4-ba62-067947633870\"},{\"content\":{\"connectorIds\":[],\"side\":\"TOP\"},\"type\":\"ConnectorPlacement.EquallySpacedRectSide\",\"uuid\":\"8d4dfadb-dd46-4985-a419-cdf5f3a788d3\"},{\"content\":{\"connectorIds\":[\"In2\"],\"side\":\"BOTTOM\"},\"type\":\"ConnectorPlacement.EquallySpacedRectSide\",\"uuid\":\"5511efcc-ad3c-4c5b-b8bc-b376c52e855b\"}]},\"type\":\"ConnectorPlacement.EquallySpacedConnector\",\"uuid\":\"a6ebe31d-a65f-4746-aee9-8fadd76d08af\"}],\"packageUris\":[\"http://schema.mathworks.com/mf0/Connector/R2020b\"],\"version\":\"1.0\"}"
  To Workspace : ToWorkspace  VariableName=Error_3142_n20  SaveFormat=Timeseries  SampleTime=-1
  To Workspace1 : ToWorkspace  VariableName=Surface_3142_n20  SaveFormat=Timeseries  SampleTime=-1
  To Workspace2 : ToWorkspace  VariableName=Response_3142_n20  SaveFormat=Timeseries  SampleTime=-1
  To Workspace3 : ToWorkspace  VariableName=Drive_3142_n20  SaveFormat=Timeseries  SampleTime=-1
  e3142 : Outport
  e3142_s : Outport  Port=2
  w+z : Outport  Port=3
  wires:
  Add3/1 -> Riemann-Liouville 2/1(In1), Subsystem1/2(De)
  Riemann-Liouville 2/1(Out1) -> Integrator/1
  Dy1/1 -> Add/1, Add3/2
  Subsystem1/2(part) -> MATLAB Function1/11(part)
  Constant/1 -> MATLAB Function1/13(phi4)
  Constant2/1 -> MATLAB Function1/12(phi3)
  w2/1 -> MATLAB Function1/6(w2)
  x2/1 -> MATLAB Function1/2(x2)
  z1/1 -> MATLAB Function1/8(z1)
  x1/1 -> MATLAB Function1/1(x1)
  Add1/1 -> Riemann-Liouville 1/1(In1)
  Riemann-Liouville 1/1(Out1) -> Integrator2/1
  "Riemann-Liouville "/1(Out1) -> Integrator1/1
  Mux/1 -> w+z/1
  Integrator1/1 -> To Workspace3/1, Mux/2  "drive"
  Add/1 -> "Riemann-Liouville "/1(In1)
  Dx3/1 -> Add/2, Add3/1
  MATLAB Function1/1(u) -> Add1/3, Add3/5
  Integrator/1 -> To Workspace/1, e3142/1, Subsystem1/1(e), Scope/1  "e"
  Dw4/1 -> Add1/1, Add3/3
  Integrator2/1 -> To Workspace2/1, Mux/1  "response"
  Dz2/1 -> Add1/2, Add3/4
  w3/1 -> MATLAB Function1/7(w3)
  Subsystem1/1(s) -> To Workspace1/1, e3142_s/1, MATLAB Function1/10(s)
  z3/1 -> MATLAB Function1/9(z3)
  x3/1 -> MATLAB Function1/3(x3)
  y1/1 -> MATLAB Function1/4(y1)
  y2/1 -> MATLAB Function1/5(y2)

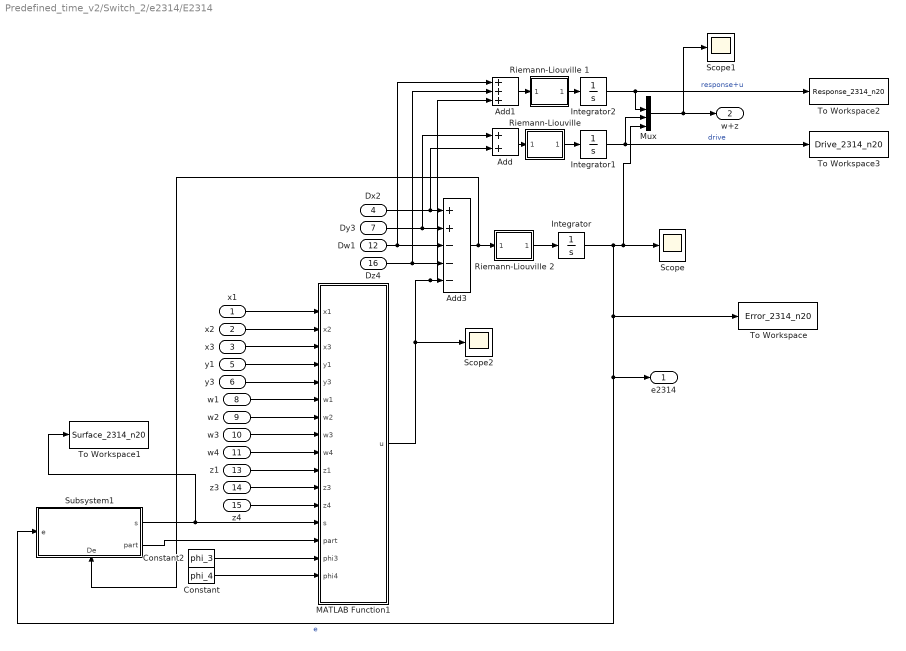
== system Predefined_time_v2/Switch_2/e2314/E2314 ==
  x1 : Inport
  x2 : Inport  Port=2
  x3 : Inport  Port=3
  Dx2 : Inport  Port=4
  y1 : Inport  Port=5
  y3 : Inport  Port=6
  Dy3 : Inport  Port=7
  w1 : Inport  Port=8
  w2 : Inport  Port=9
  w3 : Inport  Port=10
  w4 : Inport  Port=11
  Dw1 : Inport  Port=12
  z1 : Inport  Port=13
  z3 : Inport  Port=14
  z4 : Inport  Port=15
  Dz4 : Inport  Port=16
  Add : Sum
  Add1 : Sum  Inputs=+++
  Add3 : Sum  Inputs=++---
  Constant : Constant  Value=phi_4
  Constant2 : Constant  Value=phi_3
  Integrator : Integrator  InitialCondition=0.1
  Integrator1 : Integrator
  Integrator2 : Integrator
  MATLAB Function1 : MATLAB Function  TreatAsAtomicUnit=on
  Mux : Mux
  "Riemann-Liouville " : Subsystem  mask{gam=1-order, ww=[1e-3, 1e3], n=5, kF1=off, kF=Oustaloup filter}
      mask prompts: gam "Derivative order gamma"; ww "Frequency range [wb,wh]"; n "Apprixmation order"; kF1 "Is a low-pass filter required?"; kF "Filter type"
      mask init: same as Predefined_time_v2/Drive system/Riemann-Liouville 1
      mask TypeOptions kF: Oustaloup filter | Modified Oustaloup filter | Matsuda-Fujii filter
      mask Display: disp(str,'texmode','on')
  Riemann-Liouville 1 : Subsystem  mask{gam=1-order, ww=[1e-3, 1e3], n=5, kF1=off, kF=Oustaloup filter}
      mask prompts: gam "Derivative order gamma"; ww "Frequency range [wb,wh]"; n "Apprixmation order"; kF1 "Is a low-pass filter required?"; kF "Filter type"
      mask init: same as Predefined_time_v2/Drive system/Riemann-Liouville 1
      mask TypeOptions kF: Oustaloup filter | Modified Oustaloup filter | Matsuda-Fujii filter
      mask Display: disp(str,'texmode','on')
  Riemann-Liouville 2 : Subsystem  mask{gam=1-order, ww=[1e-3, 1e3], n=5, kF1=off, kF=Oustaloup filter}
      mask prompts: gam "Derivative order gamma"; ww "Frequency range [wb,wh]"; n "Apprixmation order"; kF1 "Is a low-pass filter required?"; kF "Filter type"
      mask init: same as Predefined_time_v2/Drive system/Riemann-Liouville 1
      mask TypeOptions kF: Oustaloup filter | Modified Oustaloup filter | Matsuda-Fujii filter
      mask Display: disp(str,'texmode','on')
  Scope : Scope
  Scope1 : Scope
  Scope2 : Scope
  Subsystem1 : Subsystem
      settings: PortSchema="{\"entries\":[{\"content\":{\"sides\":[{\"content\":{\"connectorIds\":[\"In1\"]},\"type\":\"ConnectorPlacement.EquallySpacedRectSide\",\"uuid\":\"1e5d287b-80a1-40a3-bd98-2fb678fb874f\"},{\"content\":{\"connectorIds\":[\"Out1\",\"Out2\"],\"side\":\"RIGHT\"},\"type\":\"ConnectorPlacement.EquallySpacedRectSide\",\"uuid\":\"9f557e7f-4584-4da4-ba62-067947633870\"},{\"content\":{\"connectorIds\":[],\"side\":\"TOP\"},\"type\":\"ConnectorPlacement.EquallySpacedRectSide\",\"uuid\":\"8d4dfadb-dd46-4985-a419-cdf5f3a788d3\"},{\"content\":{\"connectorIds\":[\"In2\"],\"side\":\"BOTTOM\"},\"type\":\"ConnectorPlacement.EquallySpacedRectSide\",\"uuid\":\"5511efcc-ad3c-4c5b-b8bc-b376c52e855b\"}]},\"type\":\"ConnectorPlacement.EquallySpacedConnector\",\"uuid\":\"a6ebe31d-a65f-4746-aee9-8fadd76d08af\"}],\"packageUris\":[\"http://schema.mathworks.com/mf0/Connector/R2020b\"],\"version\":\"1.0\"}"
  To Workspace : ToWorkspace  VariableName=Error_2314_n20  SaveFormat=Timeseries  SampleTime=-1
  To Workspace1 : ToWorkspace  VariableName=Surface_2314_n20  SaveFormat=Timeseries  SampleTime=-1
  To Workspace2 : ToWorkspace  VariableName=Response_2314_n20  SaveFormat=Timeseries  SampleTime=-1
  To Workspace3 : ToWorkspace  VariableName=Drive_2314_n20  SaveFormat=Timeseries  SampleTime=-1
  e2314 : Outport
  w+z : Outport  Port=2
  wires:
  Add3/1 -> Riemann-Liouville 2/1(In1), Subsystem1/2(De)
  Dz4/1 -> Add1/2, Add3/4
  Subsystem1/1(s) -> To Workspace1/1, MATLAB Function1/13(s)
  Dw1/1 -> Add1/1, Add3/3
  Riemann-Liouville 2/1(Out1) -> Integrator/1
  Dy3/1 -> Add/1, Add3/2
  Subsystem1/2(part) -> MATLAB Function1/14(part)
  Constant/1 -> MATLAB Function1/16(phi4)
  Constant2/1 -> MATLAB Function1/15(phi3)
  Add1/1 -> Riemann-Liouville 1/1(In1)
  Riemann-Liouville 1/1(Out1) -> Integrator2/1
  Integrator2/1 -> Mux/2, To Workspace2/1  "response+u"
  "Riemann-Liouville "/1(Out1) -> Integrator1/1
  Mux/1 -> Scope1/1, w+z/1
  Integrator1/1 -> Mux/3, To Workspace3/1  "drive"
  Add/1 -> "Riemann-Liouville "/1(In1)
  Dx2/1 -> Add/2, Add3/1
  Integrator/1 -> To Workspace/1, e2314/1, Subsystem1/1(e), Mux/4, Scope/1  "e"
  MATLAB Function1/1(u) -> Scope2/1, Add1/3, Add3/5
  z4/1 -> MATLAB Function1/12(z4)
  z1/1 -> MATLAB Function1/10(z1)
  y3/1 -> MATLAB Function1/5(y3)
  y1/1 -> MATLAB Function1/4(y1)
  x3/1 -> MATLAB Function1/3(x3)
  x2/1 -> MATLAB Function1/2(x2)
  x1/1 -> MATLAB Function1/1(x1)
  w4/1 -> MATLAB Function1/9(w4)
  w3/1 -> MATLAB Function1/8(w3)
  w2/1 -> MATLAB Function1/7(w2)
  w1/1 -> MATLAB Function1/6(w1)
  z3/1 -> MATLAB Function1/11(z3)

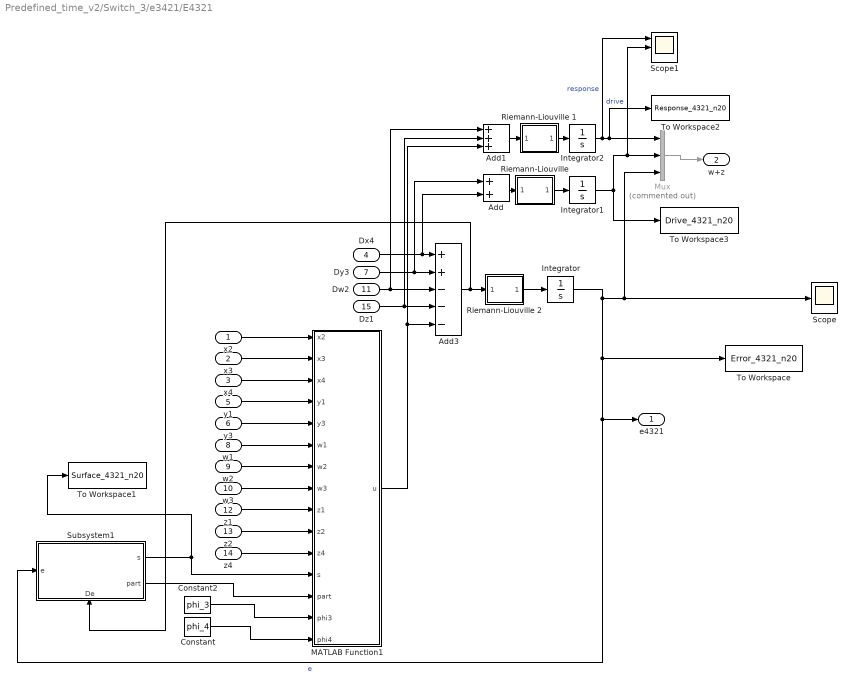
== system Predefined_time_v2/Switch_3/e3421/E4321 ==
  x2 : Inport
  x3 : Inport  Port=2
  x4 : Inport  Port=3
  Dx4 : Inport  Port=4
  y1 : Inport  Port=5
  y3 : Inport  Port=6
  Dy3 : Inport  Port=7
  w1 : Inport  Port=8
  w2 : Inport  Port=9
  w3 : Inport  Port=10
  Dw2 : Inport  Port=11
  z1 : Inport  Port=12
  z2 : Inport  Port=13
  z4 : Inport  Port=14
  Dz1 : Inport  Port=15
  Add : Sum
  Add1 : Sum  Inputs=+++
  Add3 : Sum  Inputs=++---
  Constant : Constant  Value=phi_4
  Constant2 : Constant  Value=phi_3
  Integrator : Integrator  InitialCondition=0.15
  Integrator1 : Integrator
  Integrator2 : Integrator
  MATLAB Function1 : MATLAB Function  TreatAsAtomicUnit=on
  Mux : Mux  Commented=on  Inputs=3
  "Riemann-Liouville " : Subsystem  mask{gam=1-order, ww=[1e-3, 1e3], n=5, kF1=off, kF=Oustaloup filter}
      mask prompts: gam "Derivative order gamma"; ww "Frequency range [wb,wh]"; n "Apprixmation order"; kF1 "Is a low-pass filter required?"; kF "Filter type"
      mask init: same as Predefined_time_v2/Drive system/Riemann-Liouville 1
      mask TypeOptions kF: Oustaloup filter | Modified Oustaloup filter | Matsuda-Fujii filter
      mask Display: disp(str,'texmode','on')
  Riemann-Liouville 1 : Subsystem  mask{gam=1-order, ww=[1e-3, 1e3], n=5, kF1=off, kF=Oustaloup filter}
      mask prompts: gam "Derivative order gamma"; ww "Frequency range [wb,wh]"; n "Apprixmation order"; kF1 "Is a low-pass filter required?"; kF "Filter type"
      mask init: same as Predefined_time_v2/Drive system/Riemann-Liouville 1
      mask TypeOptions kF: Oustaloup filter | Modified Oustaloup filter | Matsuda-Fujii filter
      mask Display: disp(str,'texmode','on')
  Riemann-Liouville 2 : Subsystem  mask{gam=1-order, ww=[1e-3, 1e3], n=5, kF1=off, kF=Oustaloup filter}
      mask prompts: gam "Derivative order gamma"; ww "Frequency range [wb,wh]"; n "Apprixmation order"; kF1 "Is a low-pass filter required?"; kF "Filter type"
      mask init: same as Predefined_time_v2/Drive system/Riemann-Liouville 1
      mask TypeOptions kF: Oustaloup filter | Modified Oustaloup filter | Matsuda-Fujii filter
      mask Display: disp(str,'texmode','on')
  Scope : Scope
  Scope1 : Scope  NumInputPorts=3
  Subsystem1 : Subsystem
      settings: PortSchema="{\"entries\":[{\"content\":{\"sides\":[{\"content\":{\"connectorIds\":[\"In1\"]},\"type\":\"ConnectorPlacement.EquallySpacedRectSide\",\"uuid\":\"1e5d287b-80a1-40a3-bd98-2fb678fb874f\"},{\"content\":{\"connectorIds\":[\"Out1\",\"Out2\"],\"side\":\"RIGHT\"},\"type\":\"ConnectorPlacement.EquallySpacedRectSide\",\"uuid\":\"9f557e7f-4584-4da4-ba62-067947633870\"},{\"content\":{\"connectorIds\":[],\"side\":\"TOP\"},\"type\":\"ConnectorPlacement.EquallySpacedRectSide\",\"uuid\":\"8d4dfadb-dd46-4985-a419-cdf5f3a788d3\"},{\"content\":{\"connectorIds\":[\"In2\"],\"side\":\"BOTTOM\"},\"type\":\"ConnectorPlacement.EquallySpacedRectSide\",\"uuid\":\"5511efcc-ad3c-4c5b-b8bc-b376c52e855b\"}]},\"type\":\"ConnectorPlacement.EquallySpacedConnector\",\"uuid\":\"a6ebe31d-a65f-4746-aee9-8fadd76d08af\"}],\"packageUris\":[\"http://schema.mathworks.com/mf0/Connector/R2020b\"],\"version\":\"1.0\"}"
  To Workspace : ToWorkspace  VariableName=Error_4321_n20  SaveFormat=Timeseries  SampleTime=-1
  To Workspace1 : ToWorkspace  VariableName=Surface_4321_n20  SaveFormat=Timeseries  SampleTime=-1
  To Workspace2 : ToWorkspace  VariableName=Response_4321_n20  SaveFormat=Timeseries  SampleTime=-1
  To Workspace3 : ToWorkspace  VariableName=Drive_4321_n20  SaveFormat=Timeseries  SampleTime=-1
  e4321 : Outport
  w+z : Outport  Port=2
  wires:
  Add3/1 -> Riemann-Liouville 2/1(In1), Subsystem1/2(De)
  Dz1/1 -> Add1/2, Add3/4
  Subsystem1/1(s) -> To Workspace1/1, MATLAB Function1/12(s)
  Dw2/1 -> Add1/1, Add3/3
  Riemann-Liouville 2/1(Out1) -> Integrator/1
  Dy3/1 -> Add/1, Add3/2
  Subsystem1/2(part) -> MATLAB Function1/13(part)
  Constant/1 -> MATLAB Function1/15(phi4)
  Constant2/1 -> MATLAB Function1/14(phi3)
  Add1/1 -> Riemann-Liouville 1/1(In1)
  Riemann-Liouville 1/1(Out1) -> Integrator2/1
  Integrator2/1 -> Scope1/1, To Workspace2/1, Mux/1  "response"
  "Riemann-Liouville "/1(Out1) -> Integrator1/1
  Mux/1 -> w+z/1
  Integrator1/1 -> To Workspace3/1, Scope1/2, Mux/2  "drive"
  Add/1 -> "Riemann-Liouville "/1(In1)
  Dx4/1 -> Add/2, Add3/1
  Integrator/1 -> To Workspace/1, e4321/1, Subsystem1/1(e), Mux/3, Scope/1  "e"
  MATLAB Function1/1(u) -> Add1/3, Add3/5
  z4/1 -> MATLAB Function1/11(z4)
  z1/1 -> MATLAB Function1/9(z1)
  w2/1 -> MATLAB Function1/7(w2)
  y1/1 -> MATLAB Function1/4(y1)
  x3/1 -> MATLAB Function1/2(x3)
  x2/1 -> MATLAB Function1/1(x2)
  x4/1 -> MATLAB Function1/3(x4)
  w3/1 -> MATLAB Function1/8(w3)
  z2/1 -> MATLAB Function1/10(z2)
  w1/1 -> MATLAB Function1/6(w1)
  y3/1 -> MATLAB Function1/5(y3)
